simulink model "SF051A_SnsrOffsLrng"  (R2013b)
settings: Solver=FixedStepDiscrete  SolverMode=SingleTasking  StartTime=0.0  StopTime=1  FixedStep=0.002  RelTol=1e-3
values from neighbouring files (symbols this model uses):
  ARCHGLBPRM_10MILLISEC_SEC_F32 = DataDict.Constant    [SF051A_SnsrOffsLrng_DataDict.m]
  ARCHGLBPRM_2MILLISEC_SEC_F32 = DataDict.Constant    [SF051A_SnsrOffsLrng_DataDict.m]
  ARCHGLBPRM_2PI_ULS_F32 = DataDict.Constant    [SF051A_SnsrOffsLrng_DataDict.m]
  ARCHGLBPRM_FLOATZEROTHD_ULS_F32 = DataDict.Constant    [SF051A_SnsrOffsLrng_DataDict.m]
  ARCHGLBPRM_PIOVER180_ULS_F32 = DataDict.Constant    [SF051A_SnsrOffsLrng_DataDict.m]
  CNV100MICROSECTOSEC_SECPERCNT_F32 = DataDict.Constant    [SF051A_SnsrOffsLrng_DataDict.m]
  COVRAMTRXNIT_ULS_F32 = DataDict.Constant    [SF051A_SnsrOffsLrng_DataDict.m]
  HWAGHILIM_HWDEG_F32 = DataDict.Constant    [SF051A_SnsrOffsLrng_DataDict.m]
  HWAUTHYTHD_ULS_F32 = DataDict.Constant    [SF051A_SnsrOffsLrng_DataDict.m]
  HWTQLRNGSTSLRND_CNT_U08 = DataDict.Constant    [SF051A_SnsrOffsLrng_DataDict.m]
  HWTQLRNGSTSNEGOFFS_CNT_U08 = DataDict.Constant    [SF051A_SnsrOffsLrng_DataDict.m]
  HWTQLRNGSTSNOTLRND_CNT_U08 = DataDict.Constant    [SF051A_SnsrOffsLrng_DataDict.m]
  HWTQLRNGSTSPOSOFFS_CNT_U08 = DataDict.Constant    [SF051A_SnsrOffsLrng_DataDict.m]
  HWTQLRNGSTSZEROOFFS_CNT_U08 = DataDict.Constant    [SF051A_SnsrOffsLrng_DataDict.m]
  IDYMTRX_ULS_F32 = DataDict.Constant    [SF051A_SnsrOffsLrng_DataDict.m]
  IVS10MS_ULSPERSEC_F32 = DataDict.Constant    [SF051A_SnsrOffsLrng_DataDict.m]
  LRNGFILTICON_ULS_F32 = DataDict.Constant    [SF051A_SnsrOffsLrng_DataDict.m]
  ONE_ULS_F32 = DataDict.Constant    [SF051A_SnsrOffsLrng_DataDict.m]
  SnsrOffsLrnd = DataDict.NVM    [SF051A_SnsrOffsLrng_DataDict.m]
  SnsrOffsLrngFctEna = DataDict.Calibration    [SF051A_SnsrOffsLrng_DataDict.m]
  SnsrOffsLrngHwAgLrngDrvgDstThd = DataDict.Calibration    [SF051A_SnsrOffsLrng_DataDict.m]
  SnsrOffsLrngHwAgLrngEna = DataDict.Calibration    [SF051A_SnsrOffsLrng_DataDict.m]
  SnsrOffsLrngHwAgLrngHwVelThd = DataDict.Calibration    [SF051A_SnsrOffsLrng_DataDict.m]
  SnsrOffsLrngHwAgLrngSysTqThd = DataDict.Calibration    [SF051A_SnsrOffsLrng_DataDict.m]
  SnsrOffsLrngHwAgLrngSysTqThdMed = DataDict.Calibration    [SF051A_SnsrOffsLrng_DataDict.m]
  SnsrOffsLrngHwAgLrngSysTqThdTrustd = DataDict.Calibration    [SF051A_SnsrOffsLrng_DataDict.m]
  SnsrOffsLrngHwAgLrngSysTqThdWide = DataDict.Calibration    [SF051A_SnsrOffsLrng_DataDict.m]
  SnsrOffsLrngHwAgLrngTi = DataDict.Calibration    [SF051A_SnsrOffsLrng_DataDict.m]
  SnsrOffsLrngHwAgLrngVehSpdThd = DataDict.Calibration    [SF051A_SnsrOffsLrng_DataDict.m]
  SnsrOffsLrngHwAgLrngYawOffsDbnd = DataDict.Calibration    [SF051A_SnsrOffsLrng_DataDict.m]
  SnsrOffsLrngHwAgLrngYawRateThd = DataDict.Calibration    [SF051A_SnsrOffsLrng_DataDict.m]
  SnsrOffsLrngHwAgOffsLim = DataDict.Calibration    [SF051A_SnsrOffsLrng_DataDict.m]
  SnsrOffsLrngHwTqLrngEna = DataDict.Calibration    [SF051A_SnsrOffsLrng_DataDict.m]
  SnsrOffsLrngHwTqLrngEnaTiThd = DataDict.Calibration    [SF051A_SnsrOffsLrng_DataDict.m]
  SnsrOffsLrngHwTqLrngHwAgDbnd = DataDict.Calibration    [SF051A_SnsrOffsLrng_DataDict.m]
  SnsrOffsLrngHwTqLrngHwAgThd = DataDict.Calibration    [SF051A_SnsrOffsLrng_DataDict.m]
  SnsrOffsLrngHwTqLrngHwTqThd = DataDict.Calibration    [SF051A_SnsrOffsLrng_DataDict.m]
  SnsrOffsLrngHwTqLrngHwTqZeroOffsThd = DataDict.Calibration    [SF051A_SnsrOffsLrng_DataDict.m]
  SnsrOffsLrngHwTqLrngHwVelThd = DataDict.Calibration    [SF051A_SnsrOffsLrng_DataDict.m]
  SnsrOffsLrngHwTqLrngMeasTi = DataDict.Calibration    [SF051A_SnsrOffsLrng_DataDict.m]
  SnsrOffsLrngHwTqLrngMeasTiScar = DataDict.Calibration    [SF051A_SnsrOffsLrng_DataDict.m]
  SnsrOffsLrngHwTqLrngSampleImbThd1 = DataDict.Calibration    [SF051A_SnsrOffsLrng_DataDict.m]
  SnsrOffsLrngHwTqLrngSampleImbThd2 = DataDict.Calibration    [SF051A_SnsrOffsLrng_DataDict.m]
  SnsrOffsLrngHwTqLrngSampleThd1 = DataDict.Calibration    [SF051A_SnsrOffsLrng_DataDict.m]
  SnsrOffsLrngHwTqLrngSampleThd2 = DataDict.Calibration    [SF051A_SnsrOffsLrng_DataDict.m]
  SnsrOffsLrngHwTqLrngTiWghtCoeff = DataDict.Calibration    [SF051A_SnsrOffsLrng_DataDict.m]
  SnsrOffsLrngHwTqLrngVehSpdThd = DataDict.Calibration    [SF051A_SnsrOffsLrng_DataDict.m]
  SnsrOffsLrngHwTqOffsLim = DataDict.Calibration    [SF051A_SnsrOffsLrng_DataDict.m]
  SnsrOffsLrngSampleCntForHwTqLrngRst = DataDict.Calibration    [SF051A_SnsrOffsLrng_DataDict.m]
  SnsrOffsLrngTqInpDetnPwrEstimnThd = DataDict.Calibration    [SF051A_SnsrOffsLrng_DataDict.m]
  SnsrOffsLrngTqInpDetnSinGenrAmp = DataDict.Calibration    [SF051A_SnsrOffsLrng_DataDict.m]
  SnsrOffsLrngTqInpDetnSinGenrFrq = DataDict.Calibration    [SF051A_SnsrOffsLrng_DataDict.m]
  SnsrOffsLrngTqInpDetnStg1FilGain = DataDict.Calibration    [SF051A_SnsrOffsLrng_DataDict.m]
  SnsrOffsLrngTqInpDetnStg1WinSize = DataDict.Calibration    [SF051A_SnsrOffsLrng_DataDict.m]
  SnsrOffsLrngTqInpDetnStg2FilGainCen = DataDict.Calibration    [SF051A_SnsrOffsLrng_DataDict.m]
  SnsrOffsLrngTqInpDetnStg2FilGainDwn = DataDict.Calibration    [SF051A_SnsrOffsLrng_DataDict.m]
  SnsrOffsLrngTqInpDetnStg2FilGainUp = DataDict.Calibration    [SF051A_SnsrOffsLrng_DataDict.m]
  SnsrOffsLrngTqInpDetnStg2WinSize = DataDict.Calibration    [SF051A_SnsrOffsLrng_DataDict.m]
  SnsrOffsLrngYawLrngEna = DataDict.Calibration    [SF051A_SnsrOffsLrng_DataDict.m]
  SnsrOffsLrngYawLrngHwAgThd = DataDict.Calibration    [SF051A_SnsrOffsLrng_DataDict.m]
  SnsrOffsLrngYawLrngTi = DataDict.Calibration    [SF051A_SnsrOffsLrng_DataDict.m]
  SnsrOffsLrngYawLrngYawAThd = DataDict.Calibration    [SF051A_SnsrOffsLrng_DataDict.m]
  SnsrOffsLrngYawOffsFrshTiThd = DataDict.Calibration    [SF051A_SnsrOffsLrng_DataDict.m]
  SnsrOffsLrngYawRateOffsLim = DataDict.Calibration    [SF051A_SnsrOffsLrng_DataDict.m]
  SPDCNVN_MTRPERSECPERKPH_F32 = DataDict.Constant    [SF051A_SnsrOffsLrng_DataDict.m]
  SysGlbPrmSysTqRat = DataDict.ImprtdCal    [SF051A_SnsrOffsLrng_DataDict.m]
  TISTEP10MS_MINS_F32 = DataDict.Constant    [SF051A_SnsrOffsLrng_DataDict.m]
  TQINPDETNLOGGAIN_ULS_F32 = DataDict.Constant    [SF051A_SnsrOffsLrng_DataDict.m]
  YAWELPDTIHILIM_MINS_F32 = DataDict.Constant    [SF051A_SnsrOffsLrng_DataDict.m]
  YAWRATENOISE_VEHDEGPERSEC_F32 = DataDict.Constant    [SF051A_SnsrOffsLrng_DataDict.m]
  ZERO_ULS_F32 = DataDict.Constant    [SF051A_SnsrOffsLrng_DataDict.m]
  ZEROVECT_ULS_F32 = DataDict.Constant    [SF051A_SnsrOffsLrng_DataDict.m]
undefined symbols (not defined in the file or in its folder): NvmGetErrSts1
libraries: Fil x34, NxtrLim x20, FixdToFloat x17, FloatToFixd x16, simulink x12, NxtrAbslt x12, NxtrNvM x8, NxtrMath x3
(part 10 of 12)

== system SF051A_SnsrOffsLrng/SnsrOffsLrng/SnsrOffsLrngPer2/Enable_Function/POC/Learn/BiasEstimation_ValidityCheck ==
  note: The function learned for long enough, but the average (slowly filtered)
      | system torque was excessive, indicating road crown, cross wind, etc.
  HwTqLrngSts : Inport
  ElpsdTi : Inport  Port=2
  HwPosBiasEstRaw : Inport  Port=3
  SysTqAvrg : Inport  Port=4
  Do nothing : Subsystem  TreatAsAtomicUnit=on
  HwTqAvrg_Check : Subsystem  RequirementInfo="{'linktype_rmi_doors' '0000babd (/E-STEER Core/SubSystem Specifications/Application Functions/SF051A Sensor Offset Learning)' '#SF051A_115' 'true' 'REQ:  SF051A_115' '' } %GIDa_ee7508ac_a4c4_4f2e_8fb0_f0302cd0680f"
  If : If  RequirementInfo="{'linktype_rmi_doors' '0000babd (/E-STEER Core/SubSystem Specifications/Application Functions/SF051A Sensor Offset Learning)' '#SF051A_141' 'true' 'REQ:  SF051A_141' '' } %GIDa_6ebd0502_7fd5_4cc3_a059_86ab112d7d84"  NumInputs=2  IfExpression=u1 & u2  ElseIfExpressions=u1 & ~u2
  Limit and Keep Learned Value : Subsystem  RequirementInfo={'linktype_rmi_doors' '0000babd (/E-STEER Core/SubSystem Specifications/Application Functions/SF051A Sensor Offset Learning)' '#SF051A_141' 'true' 'REQ: SF051A_141' '' } %GIDa_1f0e41ab_d12e_487c_96e6_f1739bc149ed  TreatAsAtomicUnit=on
  Reset_HwAgLrng : Subsystem  TreatAsAtomicUnit=on
  Subsystem5 : Subsystem  Description=|  mask(Copyright Information){none=on}
      | Copyright info block.                                               
      |                                                                     
      | Place copyright information at the top of every subsystem in design.
      mask prompts: none "No parameters"
      mask help: Place copyright information at the top of every subsystem in design.
      mask Display:
      | NxtrConf = 'Nexteer Confidential';
      | 
      | sys = bdroot; %handle for the current model ("system")
      | first = get_param(sys,'Created');
      | first = first(end-3:end);  %year is last four digits
      | 
      | last = get_param(sys,'LastModifiedDate');
      | if isempty(last)
      |     last = datestr(now,'yyyy');
      | else
      |     last = last(end-3:end);
      | end
      | 
      | if strcmp(first,last)
      |     fprintf('%s -- Copyright %s Nexteer',NxtrConf,first)
      | else
      |     fprintf('%s -- %s%s- %s Nexteer',NxtrConf,char(169),first,last)
      | end
  Time_Check : Subsystem
  wires:
  HwPosBiasEstRaw/1 -> Limit and Keep Learned Value/1(HwPosBiasEstRaw)
  SysTqAvrg/1 -> HwTqAvrg_Check/1(SysTqAvrg)
  HwTqAvrg_Check/1(TqVldFlg) -> If/2
  ElpsdTi/1 -> Time_Check/1(ElpsdTi)
  Time_Check/1(TiVldFlg) -> If/1
  HwTqLrngSts/1 -> HwTqAvrg_Check/2(HwTqLrngSts)
  If/1 -> Limit and Keep Learned Value/Action
  If/2 -> Reset_HwAgLrng/Action
  If/3 -> Do nothing/Action

== system SF051A_SnsrOffsLrng/SnsrOffsLrng/SnsrOffsLrngPer2/Enable_Function/POC/Learn/LPFs ==
  note: Apply slow filters to Driver + Assist Torque. After tunable period of time, this will be used to decide whether the road was flat and wind was calm (or at least averaged themselves out over the time period).
  note: Same fc for both paths
  note: Two LPF in series to achieve a less noisy estimation
  HwAgFild : Inport
  SysTqFild : Inport  Port=2
  Add1 : Sum  RequirementInfo="{'linktype_rmi_doors' '0000babd (/E-STEER Core/SubSystem Specifications/Application Functions/SF051A Sensor Offset Learning)' '#SF051A_118' 'true' 'REQ:  SF051A_118' '' } %GIDa_a9eb681f_cac0_43af_beb2_f1f51fe05355"
  FilLpUpdOutp : Fil/FilLpUpdOutp  RequirementInfo="{'linktype_rmi_doors' '0000babd (/E-STEER Core/SubSystem Specifications/Application Functions/SF051A Sensor Offset Learning)' '#SF051A_120' 'true' 'REQ:  SF051A_120' '' } %GIDa_e30aba0f_56bd_4fdb_8776_c681c8d8de47"  StVar=HwAgLrngFil1
      settings: AttributesFormatString=StVar: %<StVar>
  FilLpUpdOutp1 : Fil/FilLpUpdOutp  RequirementInfo="{'linktype_rmi_doors' '0000babd (/E-STEER Core/SubSystem Specifications/Application Functions/SF051A Sensor Offset Learning)' '#SF051A_120' 'true' 'REQ:  SF051A_120' '' } %GIDa_e1bf3bcc_7598_44e1_9e26_8397d90c3eeb"  StVar=HwAgLrngFil2
      settings: AttributesFormatString=StVar: %<StVar>
  FilLpUpdOutp2 : Fil/FilLpUpdOutp  RequirementInfo="{'linktype_rmi_doors' '0000babd (/E-STEER Core/SubSystem Specifications/Application Functions/SF051A Sensor Offset Learning)' '#SF051A_116' 'true' 'REQ:  SF051A_116' '' } %GIDa_0425a662_6a46_4ec4_80ca_4f7f05c68403"  StVar=HwAgLrngSysTqFil1
      settings: AttributesFormatString=StVar: %<StVar>
  FilLpUpdOutp3 : Fil/FilLpUpdOutp  RequirementInfo="{'linktype_rmi_doors' '0000babd (/E-STEER Core/SubSystem Specifications/Application Functions/SF051A Sensor Offset Learning)' '#SF051A_116' 'true' 'REQ:  SF051A_116' '' } %GIDa_d241de31_ede3_4c71_a352_ed2f5f77ad04"  StVar=HwAgLrngSysTqFil2
      settings: AttributesFormatString=StVar: %<StVar>
  FloatToFixd_s16_f1 : FloatToFixd/FloatToFixd_s16_f32  Param1=5
  FloatToFixd_s16_f32 : FloatToFixd/FloatToFixd_s16_f32  Param1=4
  NvmRam : DataStoreWrite  RequirementInfo="{'linktype_rmi_doors' '0000babd (/E-STEER Core/SubSystem Specifications/Application Functions/SF051A Sensor Offset Learning)' '#SF051A_119' 'true' 'REQ:  SF051A_119' '' } %GIDa_7d3fe29f_62c5_41ed_8a64_f23320f0f4e5"  DataStoreName=SnsrOffsLrnd  DataStoreElements=SnsrOffsLrnd.HwAgLrngHwAgFilSt#SnsrOffsLrnd.HwAgLrngSysTqFilSt
  Read NVMRam : DataStoreRead  RequirementInfo="{'linktype_rmi_doors' '0000babd (/E-STEER Core/SubSystem Specifications/Application Functions/SF051A Sensor Offset Learning)' '#SF051A_118' 'true' 'REQ:  SF051A_118' '' } %GIDa_3e1188c8_61c6_4a14_9b93_b71b1baf8e86"  DataStoreName=SnsrOffsLrnd  DataStoreElements=SnsrOffsLrnd.HwAgLrndTi
  Subsystem5 : Subsystem  Description=|  mask(Copyright Information){none=on}
      | Copyright info block.                                               
      |                                                                     
      | Place copyright information at the top of every subsystem in design.
      mask prompts: none "No parameters"
      mask help: Place copyright information at the top of every subsystem in design.
      mask Display:
      | NxtrConf = 'Nexteer Confidential';
      | 
      | sys = bdroot; %handle for the current model ("system")
      | first = get_param(sys,'Created');
      | first = first(end-3:end);  %year is last four digits
      | 
      | last = get_param(sys,'LastModifiedDate');
      | if isempty(last)
      |     last = datestr(now,'yyyy');
      | else
      |     last = last(end-3:end);
      | end
      | 
      | if strcmp(first,last)
      |     fprintf('%s -- Copyright %s Nexteer',NxtrConf,first)
      | else
      |     fprintf('%s -- %s%s- %s Nexteer',NxtrConf,char(169),first,last)
      | end
  Ts : Constant  RequirementInfo="{'linktype_rmi_doors' '0000babd (/E-STEER Core/SubSystem Specifications/Application Functions/SF051A Sensor Offset Learning)' '#SF051A_118' 'true' 'REQ:  SF051A_118' '' } %GIDa_d54cb801_cb5c_4254_a813_9ff94058f6aa"  Value=ARCHGLBPRM_10MILLISEC_SEC_F32
  ElpsdTi : Outport  OutDataTypeStr=single
  HwPosBiasEstRaw : Outport  Port=2
  SysTqAvrg : Outport  RequirementInfo="{'linktype_rmi_doors' '0000babd (/E-STEER Core/SubSystem Specifications/Application Functions/SF051A Sensor Offset Learning)' '#SF051A_116' 'true' 'REQ:  SF051A_116' '' } %GIDa_b3eceb47_afae_4bf7_8f18_e381e2b43915"  Port=3
  wires:
  HwAgFild/1 -> FilLpUpdOutp/1
  FilLpUpdOutp1/1 -> FloatToFixd_s16_f32/1, HwPosBiasEstRaw/1
  SysTqFild/1 -> FilLpUpdOutp2/1
  FilLpUpdOutp3/1 -> FloatToFixd_s16_f1/1, SysTqAvrg/1
  Read NVMRam/1 -> Add1/1
  Ts/1 -> Add1/2
  Add1/1 -> ElpsdTi/1  "ElpsdTi"
  FloatToFixd_s16_f32/1 -> NvmRam/1
  FloatToFixd_s16_f1/1 -> NvmRam/2
  FilLpUpdOutp/1 -> FilLpUpdOutp1/1
  FilLpUpdOutp2/1 -> FilLpUpdOutp3/1

== system SF051A_SnsrOffsLrng/SnsrOffsLrng/SnsrOffsLrngPer2/Enable_Function/POC/Learn/Subsystem5 ==

== system SF051A_SnsrOffsLrng/SnsrOffsLrng/SnsrOffsLrngPer2/Enable_Function/POC/Learning Conditions/DrivingStraight ==
  note: Calculate distance travelled. Learning conditions must be true for a minimum driving distance before learning begins.
  VehSpd : Inport  OutDataTypeStr=single
  Action Port : ActionPort  ActionType=then
  Constant : Constant  Value=ARCHGLBPRM_10MILLISEC_SEC_F32
  Constant1 : Constant  Value=SPDCNVN_MTRPERSECPERKPH_F32
  Data Store Read : DataStoreRead  DataStoreName=HwAgLrngDrvgDstPrev
  LimStat_f32 : NxtrLim/LimStat_f32  LoLim=ZERO_ULS_F32  HiLim=SnsrOffsLrngHwAgLrngDrvgDstThd
      settings: AttributesFormatString=|
      | Low Limit: %<LoLim>
      | High Limit:%<HiLim>
  Product : Product  Inputs=3  OutDataTypeStr=single  RndMeth=Zero
  Subsystem5 : Subsystem  Description=|  mask(Copyright Information){none=on}
      | Copyright info block.                                               
      |                                                                     
      | Place copyright information at the top of every subsystem in design.
      mask prompts: none "No parameters"
      mask help: Place copyright information at the top of every subsystem in design.
      mask Display:
      | NxtrConf = 'Nexteer Confidential';
      | 
      | sys = bdroot; %handle for the current model ("system")
      | first = get_param(sys,'Created');
      | first = first(end-3:end);  %year is last four digits
      | 
      | last = get_param(sys,'LastModifiedDate');
      | if isempty(last)
      |     last = datestr(now,'yyyy');
      | else
      |     last = last(end-3:end);
      | end
      | 
      | if strcmp(first,last)
      |     fprintf('%s -- Copyright %s Nexteer',NxtrConf,first)
      | else
      |     fprintf('%s -- %s%s- %s Nexteer',NxtrConf,char(169),first,last)
      | end
  Sum : Sum
  HwAgLrngDrvgDst : Outport
  wires:
  Product/1 -> Sum/1
  Constant/1 -> Product/3
  VehSpd/1 -> Product/1
  Sum/1 -> LimStat_f32/1
  Constant1/1 -> Product/2
  Data Store Read/1 -> Sum/2
  LimStat_f32/1 -> HwAgLrngDrvgDst/1

== system SF051A_SnsrOffsLrng/SnsrOffsLrng/SnsrOffsLrngPer2/Enable_Function/POC/Learning Conditions/NotDrivingStraight ==
  Action Port : ActionPort  ActionType=else
  DistanceTravelled : Constant  Value=ZERO_ULS_F32  OutDataTypeStr=single
      settings: AttributesFormatString=%<OutDataTypeStr>
  Subsystem5 : Subsystem  Description=|  mask(Copyright Information){none=on}
      | Copyright info block.                                               
      |                                                                     
      | Place copyright information at the top of every subsystem in design.
      mask prompts: none "No parameters"
      mask help: Place copyright information at the top of every subsystem in design.
      mask Display:
      | NxtrConf = 'Nexteer Confidential';
      | 
      | sys = bdroot; %handle for the current model ("system")
      | first = get_param(sys,'Created');
      | first = first(end-3:end);  %year is last four digits
      | 
      | last = get_param(sys,'LastModifiedDate');
      | if isempty(last)
      |     last = datestr(now,'yyyy');
      | else
      |     last = last(end-3:end);
      | end
      | 
      | if strcmp(first,last)
      |     fprintf('%s -- Copyright %s Nexteer',NxtrConf,first)
      | else
      |     fprintf('%s -- %s%s- %s Nexteer',NxtrConf,char(169),first,last)
      | end
  HwAgLrngDrvgDstPrev : Outport
  wires:
  DistanceTravelled/1 -> HwAgLrngDrvgDstPrev/1

== system SF051A_SnsrOffsLrng/SnsrOffsLrng/SnsrOffsLrngPer2/Enable_Function/POC/Learning Conditions/Subsystem5 ==

== system SF051A_SnsrOffsLrng/SnsrOffsLrng/SnsrOffsLrngPer2/Enable_Function/POC/Reset_HwAg_Learning/Subsystem5 ==

== system SF051A_SnsrOffsLrng/SnsrOffsLrng/SnsrOffsLrngPer2/Enable_Function/SOaC_HierarchyManager/POCEnabler/Subsystem5 ==

== system SF051A_SnsrOffsLrng/SnsrOffsLrng/SnsrOffsLrngPer2/Enable_Function/SOaC_HierarchyManager/POCResetLogic/Subsystem5 ==

== system SF051A_SnsrOffsLrng/SnsrOffsLrng/SnsrOffsLrngPer2/Enable_Function/SOaC_HierarchyManager/YOCEnabler/Subsystem5 ==

== system SF051A_SnsrOffsLrng/SnsrOffsLrng/SnsrOffsLrngPer2/Enable_Function/YOC/Do nothing/Subsystem5 ==

== system SF051A_SnsrOffsLrng/SnsrOffsLrng/SnsrOffsLrngPer2/Enable_Function/YOC/Learn/Do nothing ==
  Action Port : ActionPort  ActionType=else
  Subsystem5 : Subsystem  Description=|  mask(Copyright Information){none=on}
      | Copyright info block.                                               
      |                                                                     
      | Place copyright information at the top of every subsystem in design.
      mask prompts: none "No parameters"
      mask help: Place copyright information at the top of every subsystem in design.
      mask Display:
      | NxtrConf = 'Nexteer Confidential';
      | 
      | sys = bdroot; %handle for the current model ("system")
      | first = get_param(sys,'Created');
      | first = first(end-3:end);  %year is last four digits
      | 
      | last = get_param(sys,'LastModifiedDate');
      | if isempty(last)
      |     last = datestr(now,'yyyy');
      | else
      |     last = last(end-3:end);
      | end
      | 
      | if strcmp(first,last)
      |     fprintf('%s -- Copyright %s Nexteer',NxtrConf,first)
      | else
      |     fprintf('%s -- %s%s- %s Nexteer',NxtrConf,char(169),first,last)
      | end

== system SF051A_SnsrOffsLrng/SnsrOffsLrng/SnsrOffsLrngPer2/Enable_Function/YOC/Learn/Filter For Learning ==
  note: Two LPF in series to achieve a less noisy estimation
  YawRate : Inport
  Display : DataStoreWrite  DataStoreName=dSnsrOffsLrngYawLrngBiasEstimnRaw
  FilLpUpdOutp : Fil/FilLpUpdOutp  RequirementInfo={'linktype_rmi_doors' '0000babd (/E-STEER Core/SubSystem Specifications/Application Functions/SF051A Sensor Offset Learning)' '#SF051A_91' 'true' 'REQ: SF051A_91' '' } %GIDa_e675741c_4393_4ae0_8c11_3d9c4cd73306  StVar=YawLrngFil1
      settings: AttributesFormatString=StVar: %<StVar>
  FilLpUpdOutp1 : Fil/FilLpUpdOutp  RequirementInfo={'linktype_rmi_doors' '0000babd (/E-STEER Core/SubSystem Specifications/Application Functions/SF051A Sensor Offset Learning)' '#SF051A_91' 'true' 'REQ: SF051A_91' '' } %GIDa_c1158e21_cba4_48b8_986e_44a0cef26229  StVar=YawLrngFil2
      settings: AttributesFormatString=StVar: %<StVar>
  Subsystem5 : Subsystem  Description=|  mask(Copyright Information){none=on}
      | Copyright info block.                                               
      |                                                                     
      | Place copyright information at the top of every subsystem in design.
      mask prompts: none "No parameters"
      mask help: Place copyright information at the top of every subsystem in design.
      mask Display:
      | NxtrConf = 'Nexteer Confidential';
      | 
      | sys = bdroot; %handle for the current model ("system")
      | first = get_param(sys,'Created');
      | first = first(end-3:end);  %year is last four digits
      | 
      | last = get_param(sys,'LastModifiedDate');
      | if isempty(last)
      |     last = datestr(now,'yyyy');
      | else
      |     last = last(end-3:end);
      | end
      | 
      | if strcmp(first,last)
      |     fprintf('%s -- Copyright %s Nexteer',NxtrConf,first)
      | else
      |     fprintf('%s -- %s%s- %s Nexteer',NxtrConf,char(169),first,last)
      | end
  LrndBias : Outport
  wires:
  YawRate/1 -> FilLpUpdOutp/1
  FilLpUpdOutp1/1 -> Display/1, LrndBias/1
  FilLpUpdOutp/1 -> FilLpUpdOutp1/1

== system SF051A_SnsrOffsLrng/SnsrOffsLrng/SnsrOffsLrngPer2/Enable_Function/YOC/Learn/Subsystem5 ==

== system SF051A_SnsrOffsLrng/SnsrOffsLrng/SnsrOffsLrngPer2/Enable_Function/YOC/Learn/Update NVM RAM ==
  LrndBias : Inport
  Action Port : ActionPort  ActionType=then
  Constant1 : Constant  RequirementInfo="{'linktype_rmi_doors' '0000babd (/E-STEER Core/SubSystem Specifications/Application Functions/SF051A Sensor Offset Learning)' '#SF051A_106' 'true' 'REQ:  SF051A_106' '' } %GIDa_37485109_fb46_48dc_909d_b521f071c2b9"  Value=SnsrOffsLrngYawRateOffsLim  OutDataTypeStr=single
  Constant3 : Constant  Value=ZERO_ULS_F32  OutDataTypeStr=single
      settings: AttributesFormatString=%<OutDataTypeStr>
  Constant4 : Constant  RequirementInfo="{'linktype_rmi_doors' '0000babd (/E-STEER Core/SubSystem Specifications/Application Functions/SF051A Sensor Offset Learning)' '#SF051A_105' 'true' 'REQ:  SF051A_105' '' ; 'linktype_rmi_doors' '0000babd (/E-STEER Core/SubSystem Specifications/Application Functions/SF051A Sensor Offset Learning)' '#SF051A_104' 'true' 'REQ:  SF051A_104' '' } %GIDa_df24ee46_4669_4b46_bb68_420380373386"  Value=true  OutDataTypeStr=boolean
      settings: AttributesFormatString=%<OutDataTypeStr>
  FloatToFixd_s16_f32 : FloatToFixd/FloatToFixd_s16_f32  Param1=9
  LimDyn_f32 : NxtrLim/LimDyn_f32  RequirementInfo="{'linktype_rmi_doors' '0000babd (/E-STEER Core/SubSystem Specifications/Application Functions/SF051A Sensor Offset Learning)' '#SF051A_106' 'true' 'REQ:  SF051A_106' '' } %GIDa_6d1d6713_3cf4_46d4_89d3_eaae33798d40"
  Subsystem5 : Subsystem  Description=|  mask(Copyright Information){none=on}
      | Copyright info block.                                               
      |                                                                     
      | Place copyright information at the top of every subsystem in design.
      mask prompts: none "No parameters"
      mask help: Place copyright information at the top of every subsystem in design.
      mask Display:
      | NxtrConf = 'Nexteer Confidential';
      | 
      | sys = bdroot; %handle for the current model ("system")
      | first = get_param(sys,'Created');
      | first = first(end-3:end);  %year is last four digits
      | 
      | last = get_param(sys,'LastModifiedDate');
      | if isempty(last)
      |     last = datestr(now,'yyyy');
      | else
      |     last = last(end-3:end);
      | end
      | 
      | if strcmp(first,last)
      |     fprintf('%s -- Copyright %s Nexteer',NxtrConf,first)
      | else
      |     fprintf('%s -- %s%s- %s Nexteer',NxtrConf,char(169),first,last)
      | end
  Unary Minus : UnaryMinus  RequirementInfo="{'linktype_rmi_doors' '0000babd (/E-STEER Core/SubSystem Specifications/Application Functions/SF051A Sensor Offset Learning)' '#SF051A_106' 'true' 'REQ:  SF051A_106' '' } %GIDa_a9a854f0_810d_4d5e_9ca1_adb6c6a73d36"
  Update NVM RAM1 : DataStoreWrite  RequirementInfo="{'linktype_rmi_doors' '0000babd (/E-STEER Core/SubSystem Specifications/Application Functions/SF051A Sensor Offset Learning)' '#SF051A_91' 'true' 'REQ:  SF051A_91' '' ; 'linktype_rmi_doors' '0000babd (/E-STEER Core/SubSystem Specifications/Application Functions/SF051A Sensor Offset Learning)' '#SF051A_240' 'true' 'REQ:  SF051A_240' '' } %GIDa_01821431_abd4_4c49_acc0_aea480f79169"  DataStoreName=SnsrOffsLrnd  DataStoreElements=SnsrOffsLrnd.YawRateOffs#SnsrOffsLrnd.YawRateOffsVld#SnsrOffsLrnd.YawRateElpdTi
  wires:
  LrndBias/1 -> LimDyn_f32/1
  Constant1/1 -> LimDyn_f32/3, Unary Minus/1
  Unary Minus/1 -> LimDyn_f32/2
  LimDyn_f32/1 -> FloatToFixd_s16_f32/1
  Constant3/1 -> Update NVM RAM1/3
  Constant4/1 -> Update NVM RAM1/2
  FloatToFixd_s16_f32/1 -> Update NVM RAM1/1

== system SF051A_SnsrOffsLrng/SnsrOffsLrng/SnsrOffsLrngPer2/Enable_Function/YOC/Learning Conditions/Subsystem5 ==

== system SF051A_SnsrOffsLrng/SnsrOffsLrng/SnsrOffsLrngPer1/EnableLearning/EnablingConditions/CheckLastMeasHwPos/FalseOut_KeepRef/Subsystem5 ==

== system SF051A_SnsrOffsLrng/SnsrOffsLrng/SnsrOffsLrngPer1/EnableLearning/EnablingConditions/CheckLastMeasHwPos/TrueOut_ResetRef/Subsystem5 ==

== system SF051A_SnsrOffsLrng/SnsrOffsLrng/SnsrOffsLrngPer1/EnableLearning/Eval_Time/GetTiSpan100MicroSec32bit/No wrapping/CopyRight2 ==

== system SF051A_SnsrOffsLrng/SnsrOffsLrng/SnsrOffsLrngPer1/EnableLearning/Eval_Time/GetTiSpan100MicroSec32bit/Wrapping/CopyRight2 ==

== system SF051A_SnsrOffsLrng/SnsrOffsLrng/SnsrOffsLrngPer1/EnableLearning/Perform_TqInpDetn/Enable_PreProcessing/False_Hold/Subsystem5 ==

== system SF051A_SnsrOffsLrng/SnsrOffsLrng/SnsrOffsLrngPer1/EnableLearning/Perform_TqInpDetn/Enable_PreProcessing/Preprocessing/Do nothing ==
  Action Port : ActionPort  ActionType=else
  Subsystem5 : Subsystem  Description=|  mask(Copyright Information){none=on}
      | Copyright info block.                                               
      |                                                                     
      | Place copyright information at the top of every subsystem in design.
      mask prompts: none "No parameters"
      mask help: Place copyright information at the top of every subsystem in design.
      mask Display:
      | NxtrConf = 'Nexteer Confidential';
      | 
      | sys = bdroot; %handle for the current model ("system")
      | first = get_param(sys,'Created');
      | first = first(end-3:end);  %year is last four digits
      | 
      | last = get_param(sys,'LastModifiedDate');
      | if isempty(last)
      |     last = datestr(now,'yyyy');
      | else
      |     last = last(end-3:end);
      | end
      | 
      | if strcmp(first,last)
      |     fprintf('%s -- Copyright %s Nexteer',NxtrConf,first)
      | else
      |     fprintf('%s -- %s%s- %s Nexteer',NxtrConf,char(169),first,last)
      | end

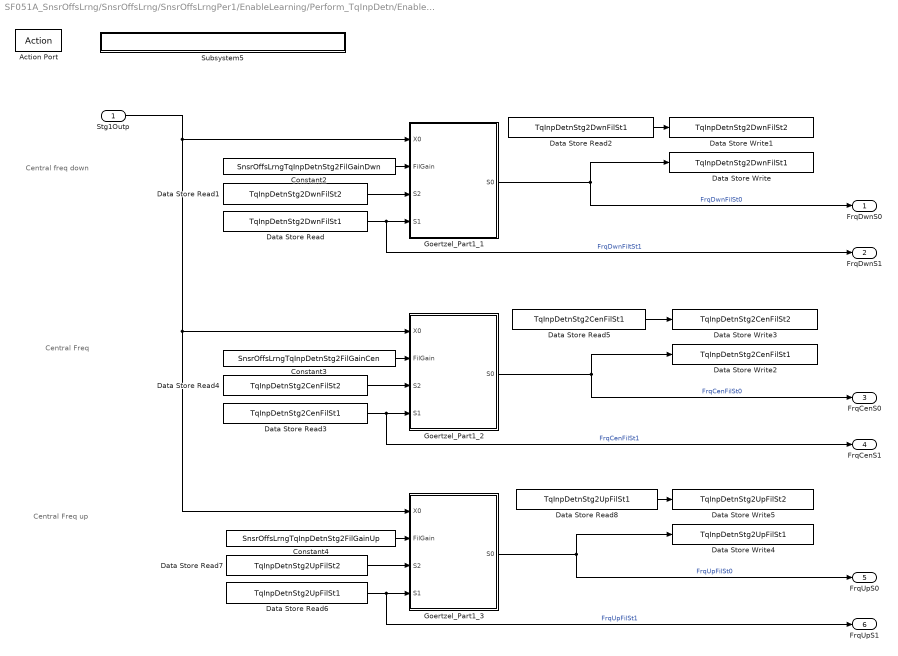
== system SF051A_SnsrOffsLrng/SnsrOffsLrng/SnsrOffsLrngPer1/EnableLearning/Perform_TqInpDetn/Enable_PreProcessing/Preprocessing/General_Goertzel ==
  note: Central Freq
  note: Central freq down
  note: Central Freq up
  Stg1Outp : Inport  OutDataTypeStr=single
  Action Port : ActionPort  ActionType=then
  Constant2 : Constant  Value=SnsrOffsLrngTqInpDetnStg2FilGainDwn
  Constant3 : Constant  Value=SnsrOffsLrngTqInpDetnStg2FilGainCen
  Constant4 : Constant  Value=SnsrOffsLrngTqInpDetnStg2FilGainUp
  Data Store Read : DataStoreRead  Priority=1  DataStoreName=TqInpDetnStg2DwnFilSt1
      settings: AttributesFormatString=priority: %<Priority>
  Data Store Read1 : DataStoreRead  Priority=1  DataStoreName=TqInpDetnStg2DwnFilSt2
  Data Store Read2 : DataStoreRead  Priority=2  DataStoreName=TqInpDetnStg2DwnFilSt1
      settings: AttributesFormatString=priority: %<Priority>
  Data Store Read3 : DataStoreRead  Priority=1  DataStoreName=TqInpDetnStg2CenFilSt1
      settings: AttributesFormatString=priority: %<Priority>
  Data Store Read4 : DataStoreRead  Priority=1  DataStoreName=TqInpDetnStg2CenFilSt2
  Data Store Read5 : DataStoreRead  Priority=2  DataStoreName=TqInpDetnStg2CenFilSt1
      settings: AttributesFormatString=priority: %<Priority>
  Data Store Read6 : DataStoreRead  Priority=1  DataStoreName=TqInpDetnStg2UpFilSt1
      settings: AttributesFormatString=priority: %<Priority>
  Data Store Read7 : DataStoreRead  Priority=1  DataStoreName=TqInpDetnStg2UpFilSt2
  Data Store Read8 : DataStoreRead  Priority=2  DataStoreName=TqInpDetnStg2UpFilSt1
      settings: AttributesFormatString=priority: %<Priority>
  Data Store Write : DataStoreWrite  Priority=3  DataStoreName=TqInpDetnStg2DwnFilSt1
      settings: AttributesFormatString=priority: %<Priority>
  Data Store Write1 : DataStoreWrite  Priority=2  DataStoreName=TqInpDetnStg2DwnFilSt2
      settings: AttributesFormatString=priority: %<Priority>
  Data Store Write2 : DataStoreWrite  Priority=3  DataStoreName=TqInpDetnStg2CenFilSt1
      settings: AttributesFormatString=priority: %<Priority>
  Data Store Write3 : DataStoreWrite  Priority=2  DataStoreName=TqInpDetnStg2CenFilSt2
      settings: AttributesFormatString=priority: %<Priority>
  Data Store Write4 : DataStoreWrite  Priority=3  DataStoreName=TqInpDetnStg2UpFilSt1
      settings: AttributesFormatString=priority: %<Priority>
  Data Store Write5 : DataStoreWrite  Priority=2  DataStoreName=TqInpDetnStg2UpFilSt2
      settings: AttributesFormatString=priority: %<Priority>
  Goertzel_Part1_1 : Subsystem  TreatAsAtomicUnit=on
      settings: RTWSystemCode=Inline
  Goertzel_Part1_2 : Subsystem  TreatAsAtomicUnit=on
      settings: RTWSystemCode=Inline
  Goertzel_Part1_3 : Subsystem  TreatAsAtomicUnit=on
      settings: RTWSystemCode=Inline
  Subsystem5 : Subsystem  Description=|  mask(Copyright Information){none=on}
      | Copyright info block.                                               
      |                                                                     
      | Place copyright information at the top of every subsystem in design.
      mask prompts: none "No parameters"
      mask help: Place copyright information at the top of every subsystem in design.
      mask Display:
      | NxtrConf = 'Nexteer Confidential';
      | 
      | sys = bdroot; %handle for the current model ("system")
      | first = get_param(sys,'Created');
      | first = first(end-3:end);  %year is last four digits
      | 
      | last = get_param(sys,'LastModifiedDate');
      | if isempty(last)
      |     last = datestr(now,'yyyy');
      | else
      |     last = last(end-3:end);
      | end
      | 
      | if strcmp(first,last)
      |     fprintf('%s -- Copyright %s Nexteer',NxtrConf,first)
      | else
      |     fprintf('%s -- %s%s- %s Nexteer',NxtrConf,char(169),first,last)
      | end
  FrqDwnS0 : Outport
  FrqDwnS1 : Outport  Port=2
  FrqCenS0 : Outport  Port=3
  FrqCenS1 : Outport  Port=4
  FrqUpS0 : Outport  Port=5
  FrqUpS1 : Outport  Port=6
  wires:
  Stg1Outp/1 -> Goertzel_Part1_3/1(X0), Goertzel_Part1_2/1(X0), Goertzel_Part1_1/1(X0)
  Goertzel_Part1_1/1(S0) -> FrqDwnS0/1, Data Store Write/1  "FrqDwnFilSt0"
  Data Store Read1/1 -> Goertzel_Part1_1/3(S2)
  Constant2/1 -> Goertzel_Part1_1/2(FilGain)
  Data Store Read2/1 -> Data Store Write1/1
  Data Store Read/1 -> FrqDwnS1/1, Goertzel_Part1_1/4(S1)  "FrqDwnFiltSt1"
  Goertzel_Part1_2/1(S0) -> FrqCenS0/1, Data Store Write2/1  "FrqCenFilSt0"
  Data Store Read4/1 -> Goertzel_Part1_2/3(S2)
  Constant3/1 -> Goertzel_Part1_2/2(FilGain)
  Data Store Read5/1 -> Data Store Write3/1
  Data Store Read3/1 -> FrqCenS1/1, Goertzel_Part1_2/4(S1)  "FrqCenFilSt1"
  Goertzel_Part1_3/1(S0) -> FrqUpS0/1, Data Store Write4/1  "FrqUpFilSt0"
  Data Store Read7/1 -> Goertzel_Part1_3/3(S2)
  Constant4/1 -> Goertzel_Part1_3/2(FilGain)
  Data Store Read8/1 -> Data Store Write5/1
  Data Store Read6/1 -> FrqUpS1/1, Goertzel_Part1_3/4(S1)  "FrqUpFilSt1"

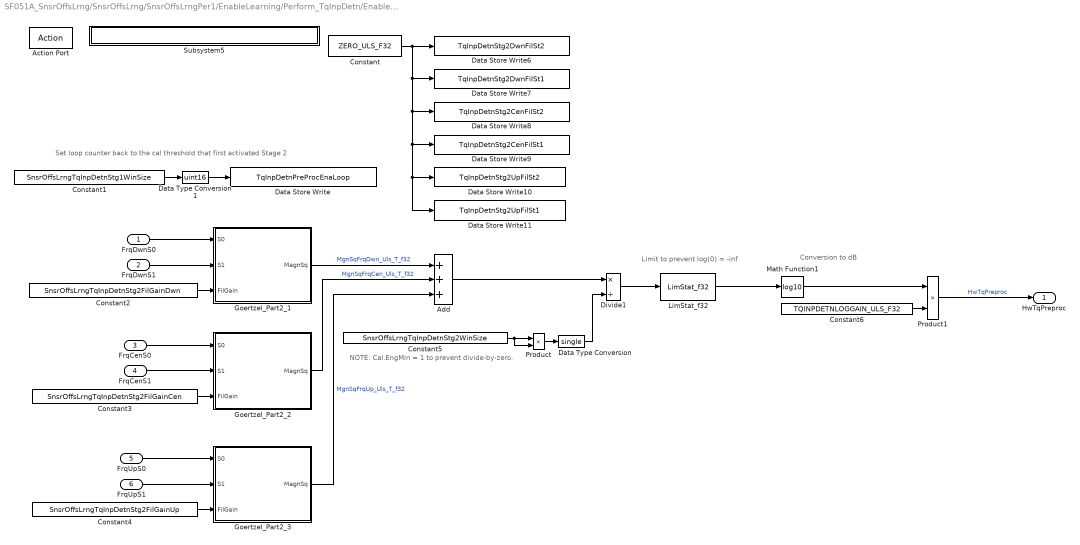
== system SF051A_SnsrOffsLrng/SnsrOffsLrng/SnsrOffsLrngPer1/EnableLearning/Perform_TqInpDetn/Enable_PreProcessing/Preprocessing/NewOut_ResetCntr ==
  note: NOTE: Cal.EngMin = 1 to prevent divide-by-zero.
  note: Set loop counter back to the cal threshold that first activated Stage 2
  note: Conversion to dB
  note: Limit to prevent log(0) = -inf
  FrqDwnS0 : Inport
  FrqDwnS1 : Inport  Port=2
  FrqCenS0 : Inport  Port=3
  FrqCenS1 : Inport  Port=4
  FrqUpS0 : Inport  Port=5
  FrqUpS1 : Inport  Port=6
  Action Port : ActionPort  ActionType=else
  Add : Sum  Inputs=+++
  Constant : Constant  Value=ZERO_ULS_F32  OutDataTypeStr=single
      settings: AttributesFormatString=%<OutDataTypeStr>
  Constant1 : Constant  Value=SnsrOffsLrngTqInpDetnStg1WinSize
  Constant2 : Constant  Value=SnsrOffsLrngTqInpDetnStg2FilGainDwn
  Constant3 : Constant  Value=SnsrOffsLrngTqInpDetnStg2FilGainCen
  Constant4 : Constant  Value=SnsrOffsLrngTqInpDetnStg2FilGainUp
  Constant5 : Constant  Value=SnsrOffsLrngTqInpDetnStg2WinSize
  Constant6 : Constant  Value=TQINPDETNLOGGAIN_ULS_F32
  Data Store Write : DataStoreWrite  DataStoreName=TqInpDetnPreProcEnaLoop
  Data Store Write10 : DataStoreWrite  DataStoreName=TqInpDetnStg2UpFilSt2
  Data Store Write11 : DataStoreWrite  DataStoreName=TqInpDetnStg2UpFilSt1
  Data Store Write6 : DataStoreWrite  DataStoreName=TqInpDetnStg2DwnFilSt2
  Data Store Write7 : DataStoreWrite  DataStoreName=TqInpDetnStg2DwnFilSt1
  Data Store Write8 : DataStoreWrite  DataStoreName=TqInpDetnStg2CenFilSt2
  Data Store Write9 : DataStoreWrite  DataStoreName=TqInpDetnStg2CenFilSt1
  Data Type Conversion : DataTypeConversion  OutDataTypeStr=single
  Data Type Conversion1 : DataTypeConversion  OutDataTypeStr=uint16
  Divide1 : Product  Inputs=*/
  Goertzel_Part2_1 : Subsystem  TreatAsAtomicUnit=on
      settings: RTWSystemCode=Inline
  Goertzel_Part2_2 : Subsystem  TreatAsAtomicUnit=on
      settings: RTWSystemCode=Inline
  Goertzel_Part2_3 : Subsystem  TreatAsAtomicUnit=on
      settings: RTWSystemCode=Inline
  LimStat_f32 : NxtrLim/LimStat_f32  LoLim=TQINPDETNLOGINPLOLIM_ULS_F32  HiLim=TQINPDETNLOGINPHILIM_ULS_F32
      settings: AttributesFormatString=|
      | Low Limit: %<LoLim>
      | High Limit:%<HiLim>
  Math Function1 : Math  Operator=log10  OutputSignalType=real  SaturateOnIntegerOverflow=on
  Product : Product
  Product1 : Product
  Subsystem5 : Subsystem  Description=|  mask(Copyright Information){none=on}
      | Copyright info block.                                               
      |                                                                     
      | Place copyright information at the top of every subsystem in design.
      mask prompts: none "No parameters"
      mask help: Place copyright information at the top of every subsystem in design.
      mask Display:
      | NxtrConf = 'Nexteer Confidential';
      | 
      | sys = bdroot; %handle for the current model ("system")
      | first = get_param(sys,'Created');
      | first = first(end-3:end);  %year is last four digits
      | 
      | last = get_param(sys,'LastModifiedDate');
      | if isempty(last)
      |     last = datestr(now,'yyyy');
      | else
      |     last = last(end-3:end);
      | end
      | 
      | if strcmp(first,last)
      |     fprintf('%s -- Copyright %s Nexteer',NxtrConf,first)
      | else
      |     fprintf('%s -- %s%s- %s Nexteer',NxtrConf,char(169),first,last)
      | end
  HwTqPreproc : Outport
  wires:
  Constant1/1 -> Data Type Conversion1/1
  Goertzel_Part2_2/1(MagnSq) -> Add/2  "MgnSqFrqCen_Uls_T_f32"
  Goertzel_Part2_3/1(MagnSq) -> Add/3  "MgnSqFrqUp_Uls_T_f32"
  Goertzel_Part2_1/1(MagnSq) -> Add/1  "MgnSqFrqDwn_Uls_T_f32"
  Product1/1 -> HwTqPreproc/1  "HwTqPreproc"
  FrqDwnS1/1 -> Goertzel_Part2_1/2(S1)
  FrqDwnS0/1 -> Goertzel_Part2_1/1(S0)
  FrqCenS1/1 -> Goertzel_Part2_2/2(S1)
  FrqCenS0/1 -> Goertzel_Part2_2/1(S0)
  FrqUpS1/1 -> Goertzel_Part2_3/2(S1)
  FrqUpS0/1 -> Goertzel_Part2_3/1(S0)
  Constant2/1 -> Goertzel_Part2_1/3(FilGain)
  Constant3/1 -> Goertzel_Part2_2/3(FilGain)
  Constant4/1 -> Goertzel_Part2_3/3(FilGain)
  Math Function1/1 -> Product1/1
  Add/1 -> Divide1/1
  Product/1 -> Data Type Conversion/1
  Divide1/1 -> LimStat_f32/1
  Constant5/1 -> Product/2, Product/1
  Data Type Conversion/1 -> Divide1/2
  Constant6/1 -> Product1/2
  Constant/1 -> Data Store Write11/1, Data Store Write10/1, Data Store Write9/1, Data Store Write8/1, Data Store Write7/1, Data Store Write6/1
  LimStat_f32/1 -> Math Function1/1
  Data Type Conversion1/1 -> Data Store Write/1

== system SF051A_SnsrOffsLrng/SnsrOffsLrng/SnsrOffsLrngPer1/EnableLearning/Perform_TqInpDetn/Enable_PreProcessing/Preprocessing/PrevOut_NoReset ==
  note: Use previous value.
  note: Save loop counter.
  note: Simulink needs to write the number of elapsed loops
      |  here instead of in the Samples counter. Otherwise the
      | write action in the NewOut_ResetCntr action block does not work.
  TqInpDetnPreProcEnaLoop : Inport
  Action Port : ActionPort  ActionType=then
  Data Store Read : DataStoreRead  DataStoreName=TqInpDetnHwTqPreProc
  Data Store Write : DataStoreWrite  DataStoreName=TqInpDetnPreProcEnaLoop
  Subsystem5 : Subsystem  Description=|  mask(Copyright Information){none=on}
      | Copyright info block.                                               
      |                                                                     
      | Place copyright information at the top of every subsystem in design.
      mask prompts: none "No parameters"
      mask help: Place copyright information at the top of every subsystem in design.
      mask Display:
      | NxtrConf = 'Nexteer Confidential';
      | 
      | sys = bdroot; %handle for the current model ("system")
      | first = get_param(sys,'Created');
      | first = first(end-3:end);  %year is last four digits
      | 
      | last = get_param(sys,'LastModifiedDate');
      | if isempty(last)
      |     last = datestr(now,'yyyy');
      | else
      |     last = last(end-3:end);
      | end
      | 
      | if strcmp(first,last)
      |     fprintf('%s -- Copyright %s Nexteer',NxtrConf,first)
      | else
      |     fprintf('%s -- %s%s- %s Nexteer',NxtrConf,char(169),first,last)
      | end
  HwTqPreproc : Outport
  wires:
  Data Store Read/1 -> HwTqPreproc/1
  TqInpDetnPreProcEnaLoop/1 -> Data Store Write/1

== system SF051A_SnsrOffsLrng/SnsrOffsLrng/SnsrOffsLrngPer1/EnableLearning/Perform_TqInpDetn/Enable_PreProcessing/Preprocessing/SampleCounter ==
  HiLim : Inport
  Add : Sum
  Data Store Read : DataStoreRead  DataStoreName=TqInpDetnPreProcEnaLoop
  LimDyn_u16 : NxtrLim/LimDyn_u16
  One_Count : Constant  OutDataTypeStr=uint16
      settings: AttributesFormatString=%<OutDataTypeStr>
  Subsystem5 : Subsystem  Description=|  mask(Copyright Information){none=on}
      | Copyright info block.                                               
      |                                                                     
      | Place copyright information at the top of every subsystem in design.
      mask prompts: none "No parameters"
      mask help: Place copyright information at the top of every subsystem in design.
      mask Display:
      | NxtrConf = 'Nexteer Confidential';
      | 
      | sys = bdroot; %handle for the current model ("system")
      | first = get_param(sys,'Created');
      | first = first(end-3:end);  %year is last four digits
      | 
      | last = get_param(sys,'LastModifiedDate');
      | if isempty(last)
      |     last = datestr(now,'yyyy');
      | else
      |     last = last(end-3:end);
      | end
      | 
      | if strcmp(first,last)
      |     fprintf('%s -- Copyright %s Nexteer',NxtrConf,first)
      | else
      |     fprintf('%s -- %s%s- %s Nexteer',NxtrConf,char(169),first,last)
      | end
  zero : Constant  Value=0  OutDataTypeStr=uint16
      settings: AttributesFormatString=%<OutDataTypeStr>
  TqInpDetnPreProcEnaLoop : Outport
  wires:
  One_Count/1 -> Add/1
  Data Store Read/1 -> Add/2
  Add/1 -> LimDyn_u16/1
  LimDyn_u16/1 -> TqInpDetnPreProcEnaLoop/1  "TqInpDetnPreProcEnaLoop"
  HiLim/1 -> LimDyn_u16/3
  zero/1 -> LimDyn_u16/2

== system SF051A_SnsrOffsLrng/SnsrOffsLrng/SnsrOffsLrngPer1/EnableLearning/Perform_TqInpDetn/Enable_PreProcessing/Preprocessing/Sliding_Goertzel_ver001 ==
  HwTqFild : Inport
  Add : Sum
  SinGen : Subsystem
  SlidingGoertzel : Subsystem
  Subsystem5 : Subsystem  Description=|  mask(Copyright Information){none=on}
      | Copyright info block.                                               
      |                                                                     
      | Place copyright information at the top of every subsystem in design.
      mask prompts: none "No parameters"
      mask help: Place copyright information at the top of every subsystem in design.
      mask Display:
      | NxtrConf = 'Nexteer Confidential';
      | 
      | sys = bdroot; %handle for the current model ("system")
      | first = get_param(sys,'Created');
      | first = first(end-3:end);  %year is last four digits
      | 
      | last = get_param(sys,'LastModifiedDate');
      | if isempty(last)
      |     last = datestr(now,'yyyy');
      | else
      |     last = last(end-3:end);
      | end
      | 
      | if strcmp(first,last)
      |     fprintf('%s -- Copyright %s Nexteer',NxtrConf,first)
      | else
      |     fprintf('%s -- %s%s- %s Nexteer',NxtrConf,char(169),first,last)
      | end
  Stg1Outp : Outport
  wires:
  SinGen/1(TqOscCmd) -> Add/2
  HwTqFild/1 -> Add/1
  SlidingGoertzel/1(Stg1Outp) -> Stg1Outp/1
  Add/1 -> SlidingGoertzel/1(HwTq)

== system SF051A_SnsrOffsLrng/SnsrOffsLrng/SnsrOffsLrngPer1/EnableLearning/Perform_TqInpDetn/Enable_PreProcessing/Preprocessing/Subsystem5 ==

== system SF051A_SnsrOffsLrng/SnsrOffsLrng/SnsrOffsLrngPer1/EnableLearning/Perform_TqInpDetn/Enable_PreProcessing/True_False/Subsystem5 ==

== system SF051A_SnsrOffsLrng/SnsrOffsLrng/SnsrOffsLrngPer1/EnableLearning/Perform_TqInpDetn/Enable_PreProcessing/True_True/Subsystem5 ==

== system SF051A_SnsrOffsLrng/SnsrOffsLrng/SnsrOffsLrngPer1/Learning/ForgettingFactor/ResetHwTqLrng/GetRefTmr100MicroSec32bit/CopyRight2 ==

== system SF051A_SnsrOffsLrng/SnsrOffsLrng/SnsrOffsLrngPer1/Learning/ValidityCheck/DecideOutputs/HwTrqNotLearnt/Subsystem5 ==

== system SF051A_SnsrOffsLrng/SnsrOffsLrng/SnsrOffsLrngPer1/Learning/ValidityCheck/DecideOutputs/HwTrqOffsetLearnt/Subsystem5 ==

== system SF051A_SnsrOffsLrng/SnsrOffsLrng/SnsrOffsLrngPer1/Learning/ValidityCheck/DecideOutputs/Pos//Neg//Zero Offset Status Selector/1_Positive HwTrq Offset ==
  Action Port : ActionPort  ActionType=then
  Constant3 : Constant  Value=HWTQLRNGSTSPOSOFFS_CNT_U08  OutDataTypeStr=uint8
  Subsystem5 : Subsystem  Description=|  mask(Copyright Information){none=on}
      | Copyright info block.                                               
      |                                                                     
      | Place copyright information at the top of every subsystem in design.
      mask prompts: none "No parameters"
      mask help: Place copyright information at the top of every subsystem in design.
      mask Display:
      | NxtrConf = 'Nexteer Confidential';
      | 
      | sys = bdroot; %handle for the current model ("system")
      | first = get_param(sys,'Created');
      | first = first(end-3:end);  %year is last four digits
      | 
      | last = get_param(sys,'LastModifiedDate');
      | if isempty(last)
      |     last = datestr(now,'yyyy');
      | else
      |     last = last(end-3:end);
      | end
      | 
      | if strcmp(first,last)
      |     fprintf('%s -- Copyright %s Nexteer',NxtrConf,first)
      | else
      |     fprintf('%s -- %s%s- %s Nexteer',NxtrConf,char(169),first,last)
      | end
  TOCStatus : Outport
  wires:
  Constant3/1 -> TOCStatus/1

== system SF051A_SnsrOffsLrng/SnsrOffsLrng/SnsrOffsLrngPer1/Learning/ValidityCheck/DecideOutputs/Pos//Neg//Zero Offset Status Selector/2_Negative HwTrq Offset ==
  Action Port : ActionPort  ActionType=elseif
  Constant3 : Constant  Value=HWTQLRNGSTSNEGOFFS_CNT_U08  OutDataTypeStr=uint8
  Subsystem5 : Subsystem  Description=|  mask(Copyright Information){none=on}
      | Copyright info block.                                               
      |                                                                     
      | Place copyright information at the top of every subsystem in design.
      mask prompts: none "No parameters"
      mask help: Place copyright information at the top of every subsystem in design.
      mask Display:
      | NxtrConf = 'Nexteer Confidential';
      | 
      | sys = bdroot; %handle for the current model ("system")
      | first = get_param(sys,'Created');
      | first = first(end-3:end);  %year is last four digits
      | 
      | last = get_param(sys,'LastModifiedDate');
      | if isempty(last)
      |     last = datestr(now,'yyyy');
      | else
      |     last = last(end-3:end);
      | end
      | 
      | if strcmp(first,last)
      |     fprintf('%s -- Copyright %s Nexteer',NxtrConf,first)
      | else
      |     fprintf('%s -- %s%s- %s Nexteer',NxtrConf,char(169),first,last)
      | end
  TOCStatus : Outport
  wires:
  Constant3/1 -> TOCStatus/1

== system SF051A_SnsrOffsLrng/SnsrOffsLrng/SnsrOffsLrngPer1/Learning/ValidityCheck/DecideOutputs/Pos//Neg//Zero Offset Status Selector/3_Zero HwTrq Offset ==
  Action Port : ActionPort  ActionType=else
  Constant3 : Constant  Value=HWTQLRNGSTSZEROOFFS_CNT_U08  OutDataTypeStr=uint8
  Subsystem5 : Subsystem  Description=|  mask(Copyright Information){none=on}
      | Copyright info block.                                               
      |                                                                     
      | Place copyright information at the top of every subsystem in design.
      mask prompts: none "No parameters"
      mask help: Place copyright information at the top of every subsystem in design.
      mask Display:
      | NxtrConf = 'Nexteer Confidential';
      | 
      | sys = bdroot; %handle for the current model ("system")
      | first = get_param(sys,'Created');
      | first = first(end-3:end);  %year is last four digits
      | 
      | last = get_param(sys,'LastModifiedDate');
      | if isempty(last)
      |     last = datestr(now,'yyyy');
      | else
      |     last = last(end-3:end);
      | end
      | 
      | if strcmp(first,last)
      |     fprintf('%s -- Copyright %s Nexteer',NxtrConf,first)
      | else
      |     fprintf('%s -- %s%s- %s Nexteer',NxtrConf,char(169),first,last)
      | end
  TOCStatus : Outport
  wires:
  Constant3/1 -> TOCStatus/1

== system SF051A_SnsrOffsLrng/SnsrOffsLrng/SnsrOffsLrngPer1/Learning/ValidityCheck/DecideOutputs/Pos//Neg//Zero Offset Status Selector/Subsystem5 ==

== system SF051A_SnsrOffsLrng/SnsrOffsLrng/SnsrOffsLrngPer2/Enable_Function/POC/Learn/BiasEstimation_ValidityCheck/Do nothing ==
  Action Port : ActionPort  ActionType=else
  Subsystem1 : Subsystem  Description=|  mask(Copyright Information){none=on}
      | Copyright info block.                                               
      |                                                                     
      | Place copyright information at the top of every subsystem in design.
      mask prompts: none "No parameters"
      mask help: Place copyright information at the top of every subsystem in design.
      mask Display:
      | NxtrConf = 'Nexteer Confidential';
      | 
      | sys = bdroot; %handle for the current model ("system")
      | first = get_param(sys,'Created');
      | first = first(end-3:end);  %year is last four digits
      | 
      | last = get_param(sys,'LastModifiedDate');
      | if isempty(last)
      |     last = datestr(now,'yyyy');
      | else
      |     last = last(end-3:end);
      | end
      | 
      | if strcmp(first,last)
      |     fprintf('%s -- Copyright %s Nexteer',NxtrConf,first)
      | else
      |     fprintf('%s -- %s%s- %s Nexteer',NxtrConf,char(169),first,last)
      | end
